simulink model "ratelim_harness"  (Simulink 4.00)
settings: Solver=FixedStepDiscrete  StartTime=0.0  StopTime=2  FixedStep=0.02  RelTol=1e-3
settings Model: RequirementInfo=9  Creator=baldrich  LastModifiedBy=baldrich  BlockReductionOpt=off  BooleanDataType=on

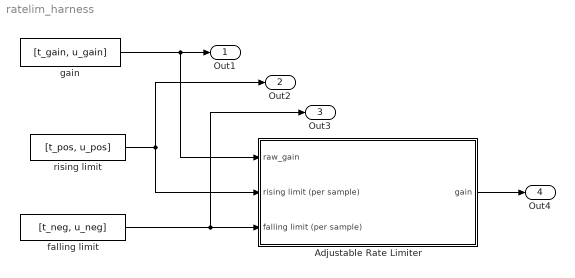
== system ratelim_harness ==
  Adjustable Rate Limiter : Subsystem
      settings: RTWFcnNameOpts=Auto  RTWFileNameOpts=Auto
  falling limit : FromWorkspace  VariableName=[t_neg, u_neg]  SampleTime=0  OutputAfterFinalValue=Extrapolation
  gain : FromWorkspace  VariableName=[t_gain, u_gain]  SampleTime=0  OutputAfterFinalValue=Extrapolation
  rising limit : FromWorkspace  VariableName=[t_pos, u_pos]  SampleTime=0  OutputAfterFinalValue=Extrapolation
  Out1 : Outport  Port=1
  Out2 : Outport  Port=2
  Out3 : Outport  Port=3
  Out4 : Outport  Port=4
  wires:
  falling limit/1 -> Adjustable Rate Limiter/3(falling limit (per sample)), Out3/1
  rising limit/1 -> Adjustable Rate Limiter/2(rising limit (per sample)), Out2/1
  gain/1 -> Out1/1, Adjustable Rate Limiter/1(raw_gain)
  Adjustable Rate Limiter/1(gain) -> Out4/1

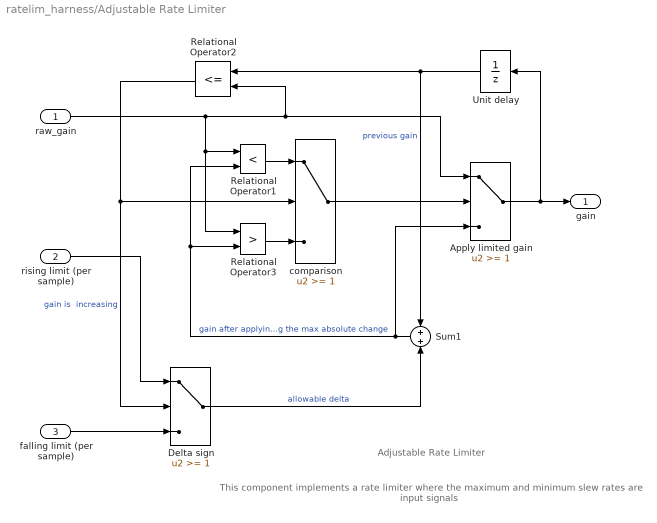
== system ratelim_harness/Adjustable Rate Limiter ==
  note: This component implements a rate limiter where the
      | maximum and minimum slew rates are input signals
  note: Adjustable Rate Limiter
  raw_gain : Inport  Port=1
  rising limit (per sample) : Inport  Port=2
  falling limit (per sample) : Inport  Port=3
  Apply limited gain : Switch  Threshold=1
  Delta sign : Switch  Threshold=1
  Relational Operator1 : RelationalOperator  Operator=<
  Relational Operator2 : RelationalOperator  Orientation=left  Operator=<=
  Relational Operator3 : RelationalOperator  Operator=>
  Sum1 : Sum  Orientation=left  Inputs=++  SaturateOnIntegerOverflow=on
  Unit delay : UnitDelay  Orientation=left  X0=0  SampleTime=.02
  comparison : Switch  Threshold=1
  gain : Outport  Port=1
  wires:
  Sum1/1 -> Apply limited gain/3, Relational Operator3/2, Relational Operator1/2  "gain after applying the max absolute change"
  comparison/1 -> Apply limited gain/2
  Relational Operator1/1 -> comparison/1
  Relational Operator3/1 -> comparison/3
  Delta sign/1 -> Sum1/2  "allowable delta"
  Relational Operator2/1 -> comparison/2, Delta sign/2  "gain is  increasing"
  falling limit (per sample)/1 -> Delta sign/3
  rising limit (per sample)/1 -> Delta sign/1
  Unit delay/1 -> Sum1/1, Relational Operator2/1  "previous gain"
  raw_gain/1 -> Relational Operator1/1, Relational Operator3/1, Relational Operator2/2, Apply limited gain/1
  Apply limited gain/1 -> Unit delay/1, gain/1
